simulink model "Analog_DSSS_WH"  (R2017a)
settings: Solver=VariableStepAuto  StartTime=0.0  StopTime=100.0  RelTol=1e-3
model workspace (MAT data in the model file):
  Amp = Simulink.Parameter
  Amp.Value = [0.5 1 1.5 2]
  Amp.DataType = 'auto'
  Amp.Dimensions = [1 4]
  FreqBase = Simulink.Parameter
  FreqBase.Value = 1.4
  FreqBase.DataType = 'auto'
  FreqBase.Dimensions = [1 1]
  FreqCode = Simulink.Parameter
  FreqCode.Value = 0.125
  FreqCode.DataType = 'auto'
  FreqCode.Dimensions = [1 1]
  Phs = Simulink.Parameter
  Phs.Value = [0 0.785398163397 1.57079632679 2.35619449019]
  Phs.DataType = 'auto'
  Phs.Dimensions = [1 4]
values from neighbouring files (symbols this model uses):
  Amp = Simulink.Parameter    [Analog_DSSS_GC_saveas.m]    (also in Analog_DSSS_WH_saveas.m)
  FreqBase = Simulink.Parameter    [Analog_DSSS_GC_saveas.m]    (also in Analog_DSSS_WH_saveas.m)
  FreqCode = Simulink.Parameter    [Analog_DSSS_GC_saveas.m]    (also in Analog_DSSS_WH_saveas.m)
  Phs = Simulink.Parameter    [Analog_DSSS_GC_saveas.m]    (also in Analog_DSSS_WH_saveas.m)
libraries: dsparch4 x4, commseqgen3 x4
settings Model: Creator=rooki  LastModifiedBy=rooki

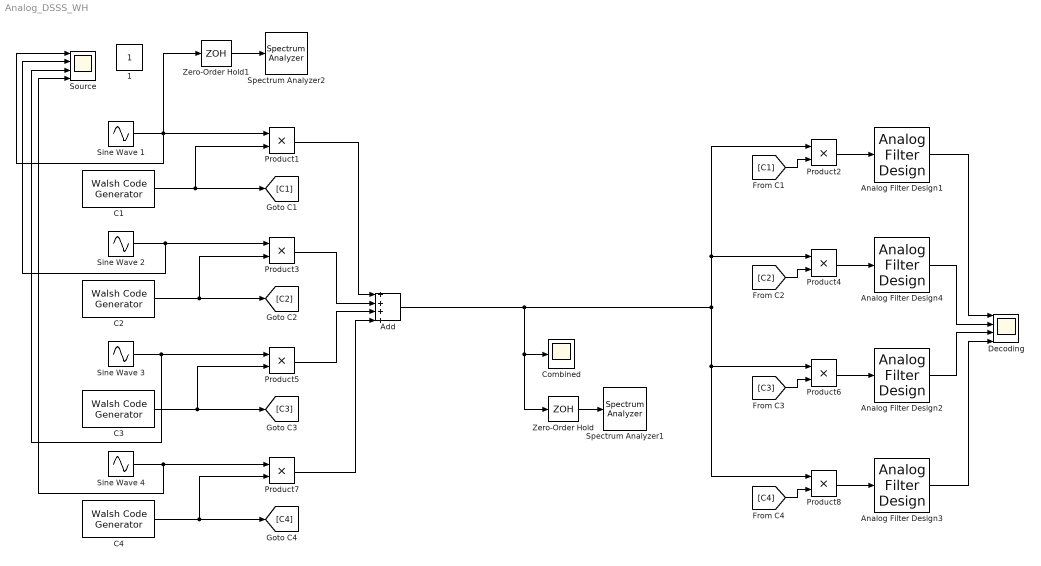
== system Analog_DSSS_WH ==
  Add : Sum  Inputs=++++
  Analog Filter Design{1..4} (4 alike) : dsparch4/Analog Filter Design  method=Butterworth  filttype=Lowpass  N=8  Wlo=2  Whi=80  Rp=2  Rs=40
  C1 : commseqgen3/Walsh Code Generator  Length=8  Index=1  SampleTime=FreqCode  SamplesPerFrame=1  OutputDataType=double  SimulateUsing=Code generation
      settings: SourceProductName=Communications System Toolbox  SourceProductBaseCode=CM
  C2 : commseqgen3/Walsh Code Generator  Length=8  Index=2  SampleTime=FreqCode  SamplesPerFrame=1  OutputDataType=double  SimulateUsing=Code generation
      settings: SourceProductName=Communications System Toolbox  SourceProductBaseCode=CM
  C3 : commseqgen3/Walsh Code Generator  Length=8  Index=3  SampleTime=FreqCode  SamplesPerFrame=1  OutputDataType=double  SimulateUsing=Code generation
      settings: SourceProductName=Communications System Toolbox  SourceProductBaseCode=CM
  C4 : commseqgen3/Walsh Code Generator  Length=8  Index=4  SampleTime=FreqCode  SamplesPerFrame=1  OutputDataType=double  SimulateUsing=Code generation
      settings: SourceProductName=Communications System Toolbox  SourceProductBaseCode=CM
  Combined : Scope
  Decoding : Scope  NumInputPorts=4
  Product{1..8} (8 alike) : Product
  Sine Wave 1 : Sin  Amplitude=Amp(1)  Frequency=FreqBase  Phase=Phs(1)  SampleTime=0
  Sine Wave 2 : Sin  Amplitude=Amp(2)  Frequency=FreqBase  Phase=Phs(2)  SampleTime=0
  Sine Wave 3 : Sin  Amplitude=Amp(3)  Frequency=FreqBase  Phase=Phs(3)  SampleTime=0
  Sine Wave 4 : Sin  Amplitude=Amp(4)  Frequency=FreqBase  Phase=Phs(4)  SampleTime=0
  Source : Scope  NumInputPorts=4
  Spectrum Analyzer1 : SpectrumAnalyzer
  Spectrum Analyzer2 : SpectrumAnalyzer
  Zero-Order Hold : ZeroOrderHold  SampleTime=1/32
  Zero-Order Hold1 : ZeroOrderHold  SampleTime=1/32
  1 : Constant  IOType=siggen
  wires:
  C1/1 -> Product1/2, [C1]
  Zero-Order Hold/1 -> Spectrum Analyzer1/1
  C2/1 -> [C2], Product3/2
  Product1/1 -> Add/1
  Product3/1 -> Add/2
  Product2/1 -> Analog Filter Design1/1
  Analog Filter Design1/1 -> Decoding/1
  Product5/1 -> Add/3
  C3/1 -> [C3], Product5/2
  Add/1 -> Zero-Order Hold/1, Combined/1, Product8/1, Product6/1, Product4/1, Product2/1
  Product7/1 -> Add/4
  C4/1 -> [C4], Product7/2
  Sine Wave 2/1 -> Source/2, Product3/1
  Sine Wave 3/1 -> Source/3, Product5/1
  Sine Wave 4/1 -> Source/4, Product7/1
  [C1] -> Product2/2
  [C2] -> Product4/2
  Product4/1 -> Analog Filter Design4/1
  Product6/1 -> Analog Filter Design2/1
  [C3] -> Product6/2
  Product8/1 -> Analog Filter Design3/1
  [C4] -> Product8/2
  Analog Filter Design4/1 -> Decoding/2
  Analog Filter Design2/1 -> Decoding/3
  Analog Filter Design3/1 -> Decoding/4
  Zero-Order Hold1/1 -> Spectrum Analyzer2/1
  Sine Wave 1/1 -> Zero-Order Hold1/1, Source/1, Product1/1
